simulink library "TBCA_lib"  (Simulink 7.5)
settings: Solver=ode45  StartTime=0.0  StopTime=10.0  RelTol=1e-3
values from neighbouring files (symbols this model uses):
  pTBCA_s_ChrgrPlgLockdTiout_C = Simulink.Parameter    [TBCA_par.m]
  pTBCA_s_ChrgrReqTiout_C = Simulink.Parameter    [TBCA_par.m]
  pTBCA_s_HandShakeTiout_C = Simulink.Parameter    [TBCA_par.m]
  pTBCA_V_ACChrgrVoltThr_C = Simulink.Parameter    [TBCA_par.m]
  pTBCA_V_DCChrgStnVoltThr_C = Simulink.Parameter    [TBCA_par.m]
undefined symbols (not defined in the file or in its folder): p_bool_False_M
libraries: BaseOperationLib_Browser x8, simulink x1
settings Model: Creator=wuaibin  LastModifiedBy=wuaibin

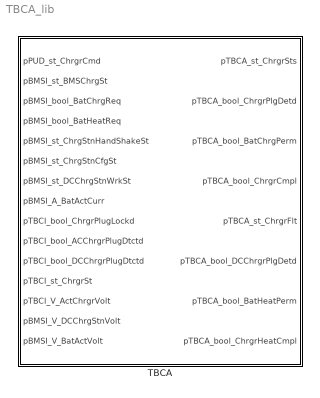
== system TBCA_lib ==
  TBCA : Subsystem  TreatAsAtomicUnit=on

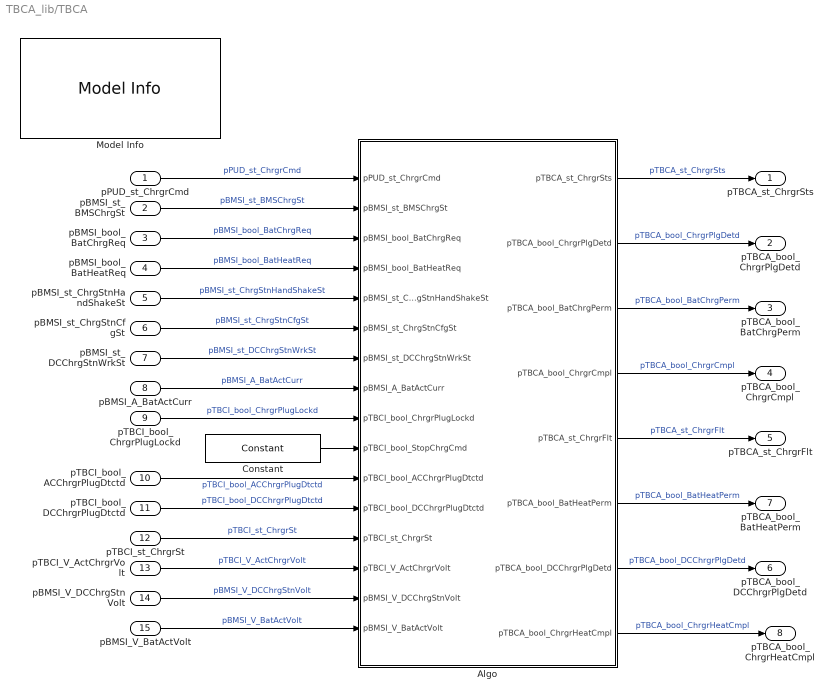
== system TBCA_lib/TBCA ==
  pPUD_st_ChrgrCmd : Inport  OutDataType=fixdt(1, 16)  OutScaling=2^0
  pBMSI_st_BMSChrgSt : Inport  Port=2  OutDataType=fixdt(1, 16)  OutScaling=2^0
  pBMSI_bool_BatChrgReq : Inport  Port=3  OutDataType=fixdt(1, 16)  OutScaling=2^0
  pBMSI_bool_BatHeatReq : Inport  Port=4  OutDataType=fixdt(1, 16)  OutScaling=2^0
  pBMSI_st_ChrgStnHandShakeSt : Inport  Port=5  OutDataType=fixdt(1, 16)  OutScaling=2^0
  pBMSI_st_ChrgStnCfgSt : Inport  Port=6  OutDataType=fixdt(1, 16)  OutScaling=2^0
  pBMSI_st_DCChrgStnWrkSt : Inport  Port=7  OutDataType=fixdt(1, 16)  OutScaling=2^0
  pBMSI_A_BatActCurr : Inport  Port=8  OutDataType=fixdt(1, 16)  OutScaling=2^0
  pTBCI_bool_ChrgrPlugLockd : Inport  Port=9  OutDataType=fixdt(1, 16)  OutScaling=2^0
  pTBCI_bool_ACChrgrPlugDtctd : Inport  Port=10  OutDataType=fixdt(1, 16)  OutScaling=2^0
  pTBCI_bool_DCChrgrPlugDtctd : Inport  Port=11  OutDataType=fixdt(1, 16)  OutScaling=2^0
  pTBCI_st_ChrgrSt : Inport  Port=12  OutDataType=fixdt(1, 16)  OutScaling=2^0
  pTBCI_V_ActChrgrVolt : Inport  Port=13  OutDataType=fixdt(1, 16)  OutScaling=2^0
  pBMSI_V_DCChrgStnVolt : Inport  Port=14  OutDataType=fixdt(1, 16)  OutScaling=2^0
  pBMSI_V_BatActVolt : Inport  Port=15  OutDataType=fixdt(1, 16)  OutScaling=2^0
  Algo : Subsystem
  Constant : BaseOperationLib_Browser/Sources&Sinks/Constant  Value=p_bool_False_M  OutMin=[]  OutMax=[]  OutDataType=fixdt(1, 16)  ConRadixGroup=Use specified scaling  OutScaling=2^0  OutDataTypeStr=Inherit: Inherit from 'Constant value'
  Model Info : simulink/Model-Wide Utilities/Model Info  SystemSampleTime=-1  InitialBlockCM=None  BlockCM=None  Frame=on  DisplayStringWithTags=Model Info\nCreated: %<Created>\nCreator: wuaibin  HorizontalTextAlignment=Center  LeftAlignmentValue=0.5  SourceBlockDiagram=HQEV_HCU  TagMaxNumber=20
  pTBCA_st_ChrgrSts : Outport  OutDataType=fixdt(1, 16)  OutScaling=2^0
  pTBCA_bool_ChrgrPlgDetd : Outport  Port=2  OutDataType=fixdt(1, 16)  OutScaling=2^0
  pTBCA_bool_BatChrgPerm : Outport  Port=3  OutDataType=fixdt(1, 16)  OutScaling=2^0
  pTBCA_bool_ChrgrCmpl : Outport  Port=4  OutDataType=fixdt(1, 16)  OutScaling=2^0
  pTBCA_st_ChrgrFlt : Outport  Port=5  OutDataType=fixdt(1, 16)  OutScaling=2^0
  pTBCA_bool_DCChrgrPlgDetd : Outport  Port=6  OutDataType=fixdt(1, 16)  OutScaling=2^0
  pTBCA_bool_BatHeatPerm : Outport  Port=7  OutDataType=fixdt(1, 16)  OutScaling=2^0
  pTBCA_bool_ChrgrHeatCmpl : Outport  Port=8  OutDataType=fixdt(1, 16)  OutScaling=2^0
  wires:
  Constant/1 -> Algo/10(pTBCI_bool_StopChrgCmd)
  pBMSI_V_DCChrgStnVolt/1 -> Algo/15(pBMSI_V_DCChrgStnVolt)  "pBMSI_V_DCChrgStnVolt"
  pTBCI_V_ActChrgrVolt/1 -> Algo/14(pTBCI_V_ActChrgrVolt)  "pTBCI_V_ActChrgrVolt"
  pBMSI_A_BatActCurr/1 -> Algo/8(pBMSI_A_BatActCurr)  "pBMSI_A_BatActCurr"
  pTBCI_st_ChrgrSt/1 -> Algo/13(pTBCI_st_ChrgrSt)  "pTBCI_st_ChrgrSt"
  Algo/8(pTBCA_bool_ChrgrHeatCmpl) -> pTBCA_bool_ChrgrHeatCmpl/1  "pTBCA_bool_ChrgrHeatCmpl"
  Algo/6(pTBCA_bool_BatHeatPerm) -> pTBCA_bool_BatHeatPerm/1  "pTBCA_bool_BatHeatPerm"
  pBMSI_st_DCChrgStnWrkSt/1 -> Algo/7(pBMSI_st_DCChrgStnWrkSt)  "pBMSI_st_DCChrgStnWrkSt"
  pBMSI_st_ChrgStnCfgSt/1 -> Algo/6(pBMSI_st_ChrgStnCfgSt)  "pBMSI_st_ChrgStnCfgSt"
  pBMSI_st_ChrgStnHandShakeSt/1 -> Algo/5(pBMSI_st_ChrgStnHandShakeSt)  "pBMSI_st_ChrgStnHandShakeSt"
  pBMSI_bool_BatHeatReq/1 -> Algo/4(pBMSI_bool_BatHeatReq)  "pBMSI_bool_BatHeatReq"
  Algo/1(pTBCA_st_ChrgrSts) -> pTBCA_st_ChrgrSts/1  "pTBCA_st_ChrgrSts"
  Algo/2(pTBCA_bool_ChrgrPlgDetd) -> pTBCA_bool_ChrgrPlgDetd/1  "pTBCA_bool_ChrgrPlgDetd"
  Algo/3(pTBCA_bool_BatChrgPerm) -> pTBCA_bool_BatChrgPerm/1  "pTBCA_bool_BatChrgPerm"
  Algo/4(pTBCA_bool_ChrgrCmpl) -> pTBCA_bool_ChrgrCmpl/1  "pTBCA_bool_ChrgrCmpl"
  Algo/5(pTBCA_st_ChrgrFlt) -> pTBCA_st_ChrgrFlt/1  "pTBCA_st_ChrgrFlt"
  pPUD_st_ChrgrCmd/1 -> Algo/1(pPUD_st_ChrgrCmd)  "pPUD_st_ChrgrCmd"
  pBMSI_st_BMSChrgSt/1 -> Algo/2(pBMSI_st_BMSChrgSt)  "pBMSI_st_BMSChrgSt"
  pTBCI_bool_ChrgrPlugLockd/1 -> Algo/9(pTBCI_bool_ChrgrPlugLockd)  "pTBCI_bool_ChrgrPlugLockd"
  pTBCI_bool_ACChrgrPlugDtctd/1 -> Algo/11(pTBCI_bool_ACChrgrPlugDtctd)  "pTBCI_bool_ACChrgrPlugDtctd"
  pBMSI_bool_BatChrgReq/1 -> Algo/3(pBMSI_bool_BatChrgReq)  "pBMSI_bool_BatChrgReq"
  pTBCI_bool_DCChrgrPlugDtctd/1 -> Algo/12(pTBCI_bool_DCChrgrPlugDtctd)  "pTBCI_bool_DCChrgrPlugDtctd"
  Algo/7(pTBCA_bool_DCChrgrPlgDetd) -> pTBCA_bool_DCChrgrPlgDetd/1  "pTBCA_bool_DCChrgrPlgDetd"
  pBMSI_V_BatActVolt/1 -> Algo/16(pBMSI_V_BatActVolt)  "pBMSI_V_BatActVolt"

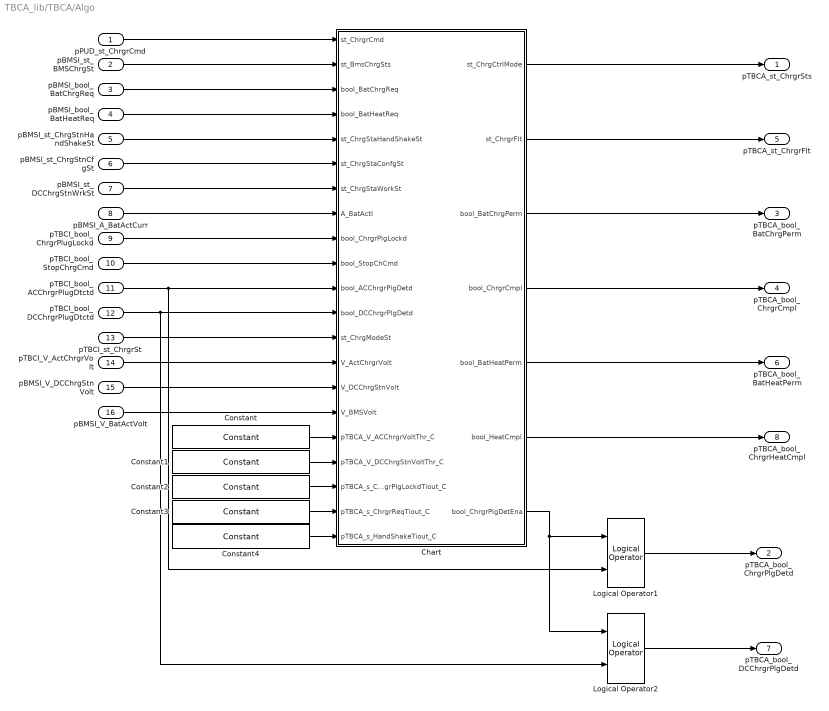
== system TBCA_lib/TBCA/Algo ==
  pPUD_st_ChrgrCmd : Inport  OutDataType=fixdt(1, 16)  OutScaling=2^0
  pBMSI_st_BMSChrgSt : Inport  Port=2  OutDataType=fixdt(1, 16)  OutScaling=2^0
  pBMSI_bool_BatChrgReq : Inport  Port=3  OutDataType=fixdt(1, 16)  OutScaling=2^0
  pBMSI_bool_BatHeatReq : Inport  Port=4  OutDataType=fixdt(1, 16)  OutScaling=2^0
  pBMSI_st_ChrgStnHandShakeSt : Inport  Port=5  OutDataType=fixdt(1, 16)  OutScaling=2^0
  pBMSI_st_ChrgStnCfgSt : Inport  Port=6  OutDataType=fixdt(1, 16)  OutScaling=2^0
  pBMSI_st_DCChrgStnWrkSt : Inport  Port=7  OutDataType=fixdt(1, 16)  OutScaling=2^0
  pBMSI_A_BatActCurr : Inport  Port=8  OutDataType=fixdt(1, 16)  OutScaling=2^0
  pTBCI_bool_ChrgrPlugLockd : Inport  Port=9  OutDataType=fixdt(1, 16)  OutScaling=2^0
  pTBCI_bool_StopChrgCmd : Inport  Port=10  OutDataType=fixdt(1, 16)  OutScaling=2^0
  pTBCI_bool_ACChrgrPlugDtctd : Inport  Port=11  OutDataType=fixdt(1, 16)  OutScaling=2^0
  pTBCI_bool_DCChrgrPlugDtctd : Inport  Port=12  OutDataType=fixdt(1, 16)  OutScaling=2^0
  pTBCI_st_ChrgrSt : Inport  Port=13  OutDataType=fixdt(1, 16)  OutScaling=2^0
  pTBCI_V_ActChrgrVolt : Inport  Port=14  OutDataType=fixdt(1, 16)  OutScaling=2^0
  pBMSI_V_DCChrgStnVolt : Inport  Port=15  OutDataType=fixdt(1, 16)  OutScaling=2^0
  pBMSI_V_BatActVolt : Inport  Port=16  OutDataType=fixdt(1, 16)  OutScaling=2^0
  Chart : Stateflow chart  TreatAsAtomicUnit=on
  Constant : BaseOperationLib_Browser/Sources&Sinks/Constant  Value=pTBCA_V_ACChrgrVoltThr_C  OutMin=[]  OutMax=[]  OutDataType=fixdt(1, 16)  ConRadixGroup=Use specified scaling  OutScaling=2^0  OutDataTypeStr=Inherit: Inherit from 'Constant value'
  Constant1 : BaseOperationLib_Browser/Sources&Sinks/Constant  Value=pTBCA_V_DCChrgStnVoltThr_C  OutMin=[]  OutMax=[]  OutDataType=fixdt(1, 16)  ConRadixGroup=Use specified scaling  OutScaling=2^0  OutDataTypeStr=Inherit: Inherit from 'Constant value'
  Constant2 : BaseOperationLib_Browser/Sources&Sinks/Constant  Value=pTBCA_s_ChrgrPlgLockdTiout_C  OutMin=[]  OutMax=[]  OutDataType=fixdt(1, 16)  ConRadixGroup=Use specified scaling  OutScaling=2^0  OutDataTypeStr=Inherit: Inherit from 'Constant value'
  Constant3 : BaseOperationLib_Browser/Sources&Sinks/Constant  Value=pTBCA_s_ChrgrReqTiout_C  OutMin=[]  OutMax=[]  OutDataType=fixdt(1, 16)  ConRadixGroup=Use specified scaling  OutScaling=2^0  OutDataTypeStr=Inherit: Inherit from 'Constant value'
  Constant4 : BaseOperationLib_Browser/Sources&Sinks/Constant  Value=pTBCA_s_HandShakeTiout_C  OutMin=[]  OutMax=[]  OutDataType=fixdt(1, 16)  ConRadixGroup=Use specified scaling  OutScaling=2^0  OutDataTypeStr=Inherit: Inherit from 'Constant value'
  Logical Operator1 : BaseOperationLib_Browser/Logic Operations Changed/Logical Operator  Operator=AND  Inputs=2  AllPortsSameDT=on  OutDataTypeMode=Specify via dialog  LogicDataType=PDT_Bool  OutDataTypeStr=PDT_Bool
  Logical Operator2 : BaseOperationLib_Browser/Logic Operations Changed/Logical Operator  Operator=AND  Inputs=2  AllPortsSameDT=on  OutDataTypeMode=Specify via dialog  LogicDataType=PDT_Bool  OutDataTypeStr=PDT_Bool
  pTBCA_st_ChrgrSts : Outport  OutDataType=fixdt(1, 16)  OutScaling=2^0
  pTBCA_bool_ChrgrPlgDetd : Outport  Port=2  OutDataType=fixdt(1, 16)  OutScaling=2^0
  pTBCA_bool_BatChrgPerm : Outport  Port=3  OutDataType=fixdt(1, 16)  OutScaling=2^0
  pTBCA_bool_ChrgrCmpl : Outport  Port=4  OutDataType=fixdt(1, 16)  OutScaling=2^0
  pTBCA_st_ChrgrFlt : Outport  Port=5  OutDataType=fixdt(1, 16)  OutScaling=2^0
  pTBCA_bool_BatHeatPerm : Outport  Port=6  OutDataType=fixdt(1, 16)  OutScaling=2^0
  pTBCA_bool_DCChrgrPlgDetd : Outport  Port=7  OutDataType=fixdt(1, 16)  OutScaling=2^0
  pTBCA_bool_ChrgrHeatCmpl : Outport  Port=8  OutDataType=fixdt(1, 16)  OutScaling=2^0
  wires:
  Constant4/1 -> Chart/21(pTBCA_s_HandShakeTiout_C)
  Constant3/1 -> Chart/20(pTBCA_s_ChrgrReqTiout_C)
  Constant2/1 -> Chart/19(pTBCA_s_ChrgrPlgLockdTiout_C)
  Constant1/1 -> Chart/18(pTBCA_V_DCChrgStnVoltThr_C)
  Constant/1 -> Chart/17(pTBCA_V_ACChrgrVoltThr_C)
  Chart/7(bool_ChrgrPlgDetEna) -> Logical Operator2/1, Logical Operator1/1
  pTBCI_bool_StopChrgCmd/1 -> Chart/10(bool_StopChCmd)
  pBMSI_V_DCChrgStnVolt/1 -> Chart/15(V_DCChrgStnVolt)
  pTBCI_V_ActChrgrVolt/1 -> Chart/14(V_ActChrgrVolt)
  pBMSI_A_BatActCurr/1 -> Chart/8(A_BatActI)
  pBMSI_st_ChrgStnCfgSt/1 -> Chart/6(st_ChrgStaConfgSt)
  pBMSI_st_ChrgStnHandShakeSt/1 -> Chart/5(st_ChrgStaHandShakeSt)
  pTBCI_st_ChrgrSt/1 -> Chart/13(st_ChrgModeSt)
  Chart/6(bool_HeatCmpl) -> pTBCA_bool_ChrgrHeatCmpl/1
  Logical Operator1/1 -> pTBCA_bool_ChrgrPlgDetd/1
  pPUD_st_ChrgrCmd/1 -> Chart/1(st_ChrgrCmd)
  Chart/1(st_ChrgCtrlMode) -> pTBCA_st_ChrgrSts/1
  Chart/2(st_ChrgrFlt) -> pTBCA_st_ChrgrFlt/1
  Chart/3(bool_BatChrgPerm) -> pTBCA_bool_BatChrgPerm/1
  Chart/4(bool_ChrgrCmpl) -> pTBCA_bool_ChrgrCmpl/1
  pBMSI_st_BMSChrgSt/1 -> Chart/2(st_BmsChrgSts)
  pTBCI_bool_ChrgrPlugLockd/1 -> Chart/9(bool_ChrgrPlgLockd)
  pBMSI_bool_BatChrgReq/1 -> Chart/3(bool_BatChrgReq)
  pTBCI_bool_ACChrgrPlugDtctd/1 -> Logical Operator1/2, Chart/11(bool_ACChrgrPlgDetd)
  pBMSI_bool_BatHeatReq/1 -> Chart/4(bool_BatHeatReq)
  pBMSI_st_DCChrgStnWrkSt/1 -> Chart/7(st_ChrgStaWorkSt)
  Chart/5(bool_BatHeatPerm) -> pTBCA_bool_BatHeatPerm/1
  pTBCI_bool_DCChrgrPlugDtctd/1 -> Logical Operator2/2, Chart/12(bool_DCChrgrPlgDetd)
  Logical Operator2/1 -> pTBCA_bool_DCChrgrPlgDetd/1
  pBMSI_V_BatActVolt/1 -> Chart/16(V_BMSVolt)

== stateflow chart TBCA/Algo/Chart ==
  state ACHeat
    state ACHeatPrecharge
      state WaitForHVON
        entry:
        st_ChrgCtrlMode = ChrgrStsTyp.CST_ACHeat_PHASE1;
      state PlugUnlocked
        entry:
        st_ChrgrFlt = FAWAlgoChrgrFltTyp.CHARGER_PLUG_LOCKING_ERR;
      state CheckPlugLocked
      state HeatingComplete
        entry:
        bool_HeatCmpl = true;
      state CheckHeatingRequest
        entry:
        bool_ChrgrPlgDetEna = true;
      (default) -> ACHeat.ACHeatPrecharge.CheckHeatingRequest
      ACHeat.ACHeatPrecharge.CheckPlugLocked -> ACHeat.ACHeatPrecharge.WaitForHVON [order 1] : [bool_ChrgrPlgLockd == true]
      ACHeat.ACHeatPrecharge.CheckPlugLocked -> ACHeat.ACHeatPrecharge.PlugUnlocked [order 2] : [bool_ChrgrPlgLockd == false && ...
          |  after(pTBCA_s_ChrgrPlgLockdTiout_C,sec)]
      ACHeat.ACHeatPrecharge.CheckHeatingRequest -> ACHeat.ACHeatPrecharge.CheckPlugLocked [order 1] : [bool_BatHeatReq == true]
      ACHeat.ACHeatPrecharge.CheckHeatingRequest -> ACHeat.ACHeatPrecharge.HeatingComplete [order 2] : [bool_BatHeatReq == false && ...
          |  after(pTBCA_s_ChrgrReqTiout_C,sec)]
    state ACHeating
      state ChargHeatPms
        entry:
        bool_ChrgrPlgDetEna = true;
        bool_BatChrgPerm = false;
        bool_BatHeatPerm = true;
      state ChargHeating1
        entry:
        st_ChrgCtrlMode = ChrgrStsTyp.CST_ACHeat_PHASE2;
      (default) -> ChargHeatPms
      ChargHeatPms -> ChargHeating1 : [st_ChrgModeSt == true]
    ACHeatPrecharge -> ACHeating : [st_ChrgrCmd == ChrgrCmdTyp.ACHeat_PHASE2]
    (default) -> ACHeatPrecharge
  state INIT
    entry:
    bool_ChrgrCmpl = false;
    bool_HeatCmpl = false;
    bool_BatChrgPerm = false;
    bool_BatHeatPerm = false;
    bool_ChrgrPlgDetEna = false;
  state DCChrg
    state DCChrgOn
      state DCCharging
        state DCChrging
          entry:
          st_ChrgCtrlMode = ChrgrStsTyp.CST_DCChrg_PHASE2;
        state DCChrgPerm
          entry:
          bool_ChrgrPlgDetEna = true;
          bool_BatHeatPerm = false;
          bool_BatChrgPerm = true;
        (default) -> DCChrgPerm
        DCChrgPerm -> DCChrging : [st_ChrgStaWorkSt == true || ...
            | V_DCChrgStnVolt >= pTBCA_V_DCChrgStnVoltThr_C]
      state DCChrgPrecharge
        state CheckChargingRequest
          entry:
          bool_ChrgrPlgDetEna = true;
        state CheckPlugLocked
        state ChargigComplete
          entry:
          bool_ChrgrCmpl = true;
        state ChrgStationHand
        state WaitForDCChrgON
          entry:
          st_ChrgCtrlMode = ChrgrStsTyp.CST_DCChrg_PHASE1;
        state HandShakeError
          entry:
          st_ChrgrFlt = FAWAlgoChrgrFltTyp.CHARGER_HANDSHAKE_ERR;
        state PlugUnlocked
          entry:
          st_ChrgrFlt = FAWAlgoChrgrFltTyp.CHARGER_PLUG_LOCKING_ERR;
        (default) -> DCChrg.DCChrgOn.DCChrgPrecharge.CheckChargingRequest
        DCChrg.DCChrgOn.DCChrgPrecharge.CheckChargingRequest -> DCChrg.DCChrgOn.DCChrgPrecharge.ChargigComplete [order 2] : [bool_BatChrgReq == false && ...
            |  after(pTBCA_s_ChrgrReqTiout_C,sec)]
        DCChrg.DCChrgOn.DCChrgPrecharge.CheckChargingRequest -> DCChrg.DCChrgOn.DCChrgPrecharge.CheckPlugLocked [order 1] : [bool_BatChrgReq == true]
        DCChrg.DCChrgOn.DCChrgPrecharge.CheckPlugLocked -> DCChrg.DCChrgOn.DCChrgPrecharge.PlugUnlocked [order 2] : [bool_ChrgrPlgLockd == false && ...
            |  after(pTBCA_s_ChrgrPlgLockdTiout_C,sec)]
        DCChrg.DCChrgOn.DCChrgPrecharge.CheckPlugLocked -> DCChrg.DCChrgOn.DCChrgPrecharge.ChrgStationHand [order 1] : [bool_ChrgrPlgLockd == true]
        DCChrg.DCChrgOn.DCChrgPrecharge.ChrgStationHand -> DCChrg.DCChrgOn.DCChrgPrecharge.HandShakeError [order 2] : [st_ChrgStaHandShakeSt == ChrgHandShakeTyp.shake_Success  && ...
            |  after(pTBCA_s_HandShakeTiout_C,sec)]
        DCChrg.DCChrgOn.DCChrgPrecharge.ChrgStationHand -> DCChrg.DCChrgOn.DCChrgPrecharge.WaitForDCChrgON [order 1] : [st_ChrgStaHandShakeSt == ChrgHandShakeTyp.shake_Success]
      (default) -> DCChrgPrecharge
      DCChrgPrecharge -> DCCharging : [st_ChrgrCmd == ChrgrCmdTyp.DCChrg_PHASE2]
    state DCChrgingFinish
      entry:
      bool_BatChrgPerm = false;
      bool_ChrgrCmpl = true;
    DCChrgOn -> DCChrgingFinish : [st_BmsChrgSts == BMSChrgStsTyp.BMS_CH_FINISH]
    (default) -> DCChrgOn
  state STOP
    entry:
    bool_BatChrgPerm = false;
    bool_BatHeatPerm = false;
    bool_ChrgrPlgDetEna = false;
    state CST_STOP
      entry:
      st_ChrgCtrlMode = ChrgrStsTyp.CST_STOP;
    (default) -> CST_STOP
  state ACChrg
    state ACChrgOn
      state ACCharging
        state ACChargePerm
          entry:
          bool_ChrgrPlgDetEna = true;
          bool_BatChrgPerm = true;
          bool_BatHeatPerm = false;
        state ACCharge
          entry:
          st_ChrgCtrlMode = ChrgrStsTyp.CST_ACChrg_PHASE2;
        (default) -> ACChargePerm
        ACChargePerm -> ACCharge : [st_ChrgModeSt == true]
      state ACChrgPrecharge
        state PlugUnlocked
          entry:
          st_ChrgrFlt = FAWAlgoChrgrFltTyp.CHARGER_PLUG_LOCKING_ERR;
        state CheckChargingRequest
          entry:
          bool_ChrgrPlgDetEna = true;
        state CheckPlugLocked
        state ChargigComplete
          entry:
          bool_ChrgrCmpl = true;
        state WaitForHVON
          entry:
          st_ChrgCtrlMode = ChrgrStsTyp.CST_ACChrg_PHASE1;
        ACChrg.ACChrgOn.ACChrgPrecharge.CheckChargingRequest -> ACChrg.ACChrgOn.ACChrgPrecharge.CheckPlugLocked [order 1] : [bool_BatChrgReq == true]
        ACChrg.ACChrgOn.ACChrgPrecharge.CheckPlugLocked -> ACChrg.ACChrgOn.ACChrgPrecharge.WaitForHVON [order 1] : [bool_ChrgrPlgLockd == true]
        ACChrg.ACChrgOn.ACChrgPrecharge.CheckPlugLocked -> ACChrg.ACChrgOn.ACChrgPrecharge.PlugUnlocked [order 2] : [bool_ChrgrPlgLockd == false && ...
            |  after(pTBCA_s_ChrgrPlgLockdTiout_C,sec)]
        (default) -> ACChrg.ACChrgOn.ACChrgPrecharge.CheckChargingRequest
        ACChrg.ACChrgOn.ACChrgPrecharge.CheckChargingRequest -> ACChrg.ACChrgOn.ACChrgPrecharge.ChargigComplete [order 2] : [bool_BatChrgReq == false && ...
            |  after(pTBCA_s_ChrgrReqTiout_C,sec)]
      ACChrgPrecharge -> ACCharging : [st_ChrgrCmd == ChrgrCmdTyp.ACChrg_PHASE2]
      (default) -> ACChrgPrecharge
    state ChargingFinish
      entry:
      bool_BatChrgPerm = false;
      bool_ChrgrCmpl = true;
    ACChrgOn -> ChargingFinish : [ st_BmsChrgSts == BMSChrgStsTyp.BMS_CH_FINISH]
    (default) -> ACChrgOn
  state DCHeat
    state DCHeating
      state DCChrgHeating
        entry:
        st_ChrgCtrlMode = ChrgrStsTyp.CST_DCHeat_PHASE2;
      state DCChrgHeatPerm
        entry:
        bool_ChrgrPlgDetEna = true;
        bool_BatChrgPerm = false;
        bool_BatHeatPerm = true;
      DCChrgHeatPerm -> DCChrgHeating : [st_ChrgStaWorkSt == true || ...
          | V_DCChrgStnVolt >= pTBCA_V_DCChrgStnVoltThr_C]
      (default) -> DCChrgHeatPerm
    state DCHeatPrecharge
      state WaitForDCChrgON
        entry:
        st_ChrgCtrlMode = ChrgrStsTyp.CST_DCHeat_PHASE1;
      state CheckPlugLocked
      state PlugUnlocked
        entry:
        st_ChrgrFlt = FAWAlgoChrgrFltTyp.CHARGER_PLUG_LOCKING_ERR;
      state ChrgStationHand
      state HandShakeError
        entry:
        st_ChrgrFlt = FAWAlgoChrgrFltTyp.CHARGER_HANDSHAKE_ERR;
      state CheckHeatingRequest
        entry:
        bool_ChrgrPlgDetEna = true;
      state HeatingComplete
        entry:
        bool_HeatCmpl = true;
      (default) -> DCHeat.DCHeatPrecharge.CheckHeatingRequest
      DCHeat.DCHeatPrecharge.CheckHeatingRequest -> DCHeat.DCHeatPrecharge.HeatingComplete [order 2] : [bool_BatHeatReq == false && ...
          |  after(pTBCA_s_ChrgrReqTiout_C,sec)]
      DCHeat.DCHeatPrecharge.CheckHeatingRequest -> DCHeat.DCHeatPrecharge.CheckPlugLocked [order 1] : [bool_BatHeatReq == true]
      DCHeat.DCHeatPrecharge.CheckPlugLocked -> DCHeat.DCHeatPrecharge.PlugUnlocked [order 2] : [bool_ChrgrPlgLockd == false && ...
          |  after(pTBCA_s_ChrgrPlgLockdTiout_C,sec)]
      DCHeat.DCHeatPrecharge.CheckPlugLocked -> DCHeat.DCHeatPrecharge.ChrgStationHand [order 1] : [bool_ChrgrPlgLockd == true]
      DCHeat.DCHeatPrecharge.ChrgStationHand -> DCHeat.DCHeatPrecharge.HandShakeError [order 2] : [st_ChrgStaHandShakeSt == ChrgHandShakeTyp.shake_Success && ...
          |  after(pTBCA_s_HandShakeTiout_C,sec)]
      DCHeat.DCHeatPrecharge.ChrgStationHand -> DCHeat.DCHeatPrecharge.WaitForDCChrgON [order 1] : [st_ChrgStaHandShakeSt == ChrgHandShakeTyp.shake_Success]
    DCHeatPrecharge -> DCHeating : [st_ChrgrCmd == ChrgrCmdTyp.DCHeat_PHASE2]
    (default) -> DCHeatPrecharge
  ACHeat -> STOP : [st_ChrgrCmd == ChrgrCmdTyp.STOP || bool_StopChCmd || bool_HeatCmpl || ...
      | bool_BatHeatReq == false]
  INIT -> STOP [order 5] : [st_ChrgrCmd == ChrgrCmdTyp.STOP]
  STOP -> DCChrg [order 4] : [st_ChrgrCmd == ChrgrCmdTyp.DCChrg_PHASE1]
  INIT -> DCChrg [order 3] : [st_ChrgrCmd == ChrgrCmdTyp.DCChrg_PHASE1]
  STOP -> DCHeat [order 3] : [st_ChrgrCmd == ChrgrCmdTyp.DCHeat_PHASE1]
  (default) -> INIT
  INIT -> ACHeat [order 1] : [st_ChrgrCmd == ChrgrCmdTyp.ACHeat_PHASE1]
  INIT -> ACChrg [order 4] : [st_ChrgrCmd == ChrgrCmdTyp.ACChrg_PHASE1]
  ACChrg -> STOP : [st_ChrgrCmd == ChrgrCmdTyp.STOP || bool_StopChCmd || bool_ChrgrCmpl]
  INIT -> DCHeat [order 2] : [st_ChrgrCmd == ChrgrCmdTyp.DCHeat_PHASE1]
  DCHeat -> STOP : [st_ChrgrCmd == ChrgrCmdTyp.STOP || bool_StopChCmd || bool_HeatCmpl || ...
      | bool_BatHeatReq == false]
  DCChrg -> STOP : [st_ChrgrCmd == ChrgrCmdTyp.STOP || bool_StopChCmd || bool_ChrgrCmpl]
  STOP -> ACHeat [order 1] : [st_ChrgrCmd == ChrgrCmdTyp.ACHeat_PHASE1]
  STOP -> ACChrg [order 2] : [st_ChrgrCmd == ChrgrCmdTyp.ACChrg_PHASE1]
  data: st_ChrgrCmd input double; st_BmsChrgSts input double; bool_BatChrgReq input double; st_ChrgCtrlMode output uint8; st_ChrgrFlt output uint32; bool_BatChrgPerm output boolean; bool_ChrgrCmpl output boolean; bool_BatHeatPerm output boolean; bool_HeatCmpl output boolean; bool_BatHeatReq input double; bool_ChrgrPlgDetEna output boolean; st_ChrgStaHandShakeSt input double; st_ChrgStaConfgSt input double; st_ChrgStaWorkSt input double; A_BatActI input double; bool_ChrgrPlgLockd input double; bool_StopChCmd input double; bool_ACChrgrPlgDetd input double; bool_DCChrgrPlgDetd input double; st_ChrgModeSt input double; V_ActChrgrVolt input double; V_DCChrgStnVolt input double; V_BMSVolt input double; pTBCA_V_ACChrgrVoltThr_C input double; pTBCA_V_DCChrgStnVoltThr_C input double; pTBCA_s_ChrgrPlgLockdTiout_C input double; pTBCA_s_ChrgrReqTiout_C input double; pTBCA_s_HandShakeTiout_C input double
